simulink model "HANcoder_E407_TTA_Controller_v3_2"  (R2018b)
settings: Solver=FixedStepDiscrete  StartTime=0.0  StopTime=1  FixedStep=0.01  RelTol=1e-3
PreLoadFcn:
  | librarySetup
  | eval([bdroot,'_startup']) %Calling [modelName]_startup.m
undefined symbols (not defined in the file): A0, A1, A2, A3, A4, Backup_Board, basic_cycle_duration_bc0, basic_cycle_duration_bc1, comm_delay_estimation1, comm_delay_estimation2, COMM_Period, COMM_Phase1, COMM_Phase2, COMM_Phase_init1, COMM_Phase_init2, COMP_duration, CON2, CON4, Controller1_Board, Controller2_Board, Controller3_Board, D10, D12, D13, D8, D9, delta_a_set, delta_f_set, delta_max, delta_min, delta_precision, e_width, frequency_IRQ, HANtuneOverride, hardware_granularity, I_a, I_f, idle_time_init, Input_Gen_Board, LA_Clock_Gr, LA_COMM_dly, LA_COMM_Err, LA_E_Desync, LA_MEX_Flag, LA_Task_Act, m_v, Master_Role, matrix_cycle_duration, matrix_rows, max_desync, max_num_msgs_CAN1, max_num_msgs_CAN2, min_desync, OutControl1_ID, OutControl2_ID, OutEmulator_ID, R_al, R_ar, R_fl, R_fr ... (+80)
libraries: hdlsllib x434, HANcoder_STM32_Target x28, simulink x3, simulink_extras x1
(part 5 of 31)

== system HANcoder_E407_TTA_Controller_v3_2/HANcoder STM32 Target - E407-STM32 algorithm/TTA CAN System/CAN2 Recieve/RxID_CAN/SetValues_ID_CAN/CAN receive1 ==
  In1 : Inport
  Enabled Subsystem : Subsystem  TreatAsAtomicUnit=on
  S-Function : M-S-Function  FunctionName=sfcn_can_receive  Parameters=tsamp, canBus, outputNumber, dataType, byteOrder
  Out1 : Outport
  Out2 : Outport  Port=2
  Out3 : Outport  Port=3
  Out4 : Outport  Port=4
  Out5 : Outport  Port=5
  Out6 : Outport  Port=6
  Out7 : Outport  Port=7
  Out8 : Outport  Port=8
  Out9 : Outport  Port=9
  wires:
  S-Function/9 -> Enabled Subsystem/8(In8)
  S-Function/4 -> Enabled Subsystem/3(In3)
  S-Function/5 -> Enabled Subsystem/4(In4)
  S-Function/8 -> Enabled Subsystem/7(In7)
  S-Function/7 -> Enabled Subsystem/6(In6)
  S-Function/6 -> Enabled Subsystem/5(In5)
  Enabled Subsystem/8(Out8) -> Out9/1
  Enabled Subsystem/7(Out7) -> Out8/1
  Enabled Subsystem/6(Out6) -> Out7/1
  Enabled Subsystem/5(Out5) -> Out6/1
  Enabled Subsystem/4(Out4) -> Out5/1
  Enabled Subsystem/3(Out3) -> Out4/1
  Enabled Subsystem/2(Out2) -> Out3/1
  Enabled Subsystem/1(Out1) -> Out2/1
  S-Function/3 -> Enabled Subsystem/2(In2)
  S-Function/2 -> Enabled Subsystem/1(In1)
  S-Function/1 -> Out1/1, Enabled Subsystem/Enable
  In1/1 -> S-Function/1

== system HANcoder_E407_TTA_Controller_v3_2/HANcoder STM32 Target - E407-STM32 algorithm/TTA CAN System/CAN2 Recieve/RxID_CAN/Sync_ID_CAN/CAN receive1 ==
  In1 : Inport
  Enabled Subsystem : Subsystem  TreatAsAtomicUnit=on
  S-Function : M-S-Function  FunctionName=sfcn_can_receive  Parameters=tsamp, canBus, outputNumber, dataType, byteOrder
  Out1 : Outport
  Out2 : Outport  Port=2
  Out3 : Outport  Port=3
  Out4 : Outport  Port=4
  Out5 : Outport  Port=5
  Out6 : Outport  Port=6
  Out7 : Outport  Port=7
  Out8 : Outport  Port=8
  Out9 : Outport  Port=9
  wires:
  S-Function/9 -> Enabled Subsystem/8(In8)
  S-Function/4 -> Enabled Subsystem/3(In3)
  S-Function/5 -> Enabled Subsystem/4(In4)
  S-Function/8 -> Enabled Subsystem/7(In7)
  S-Function/7 -> Enabled Subsystem/6(In6)
  S-Function/6 -> Enabled Subsystem/5(In5)
  Enabled Subsystem/8(Out8) -> Out9/1
  Enabled Subsystem/7(Out7) -> Out8/1
  Enabled Subsystem/6(Out6) -> Out7/1
  Enabled Subsystem/5(Out5) -> Out6/1
  Enabled Subsystem/4(Out4) -> Out5/1
  Enabled Subsystem/3(Out3) -> Out4/1
  Enabled Subsystem/2(Out2) -> Out3/1
  Enabled Subsystem/1(Out1) -> Out2/1
  S-Function/3 -> Enabled Subsystem/2(In2)
  S-Function/2 -> Enabled Subsystem/1(In1)
  S-Function/1 -> Out1/1, Enabled Subsystem/Enable
  In1/1 -> S-Function/1

== system HANcoder_E407_TTA_Controller_v3_2/HANcoder STM32 Target - E407-STM32 algorithm/TTA CAN System/CAN2 Recieve/RxID_CAN/Vote1_ID_CAN/CAN receive1 ==
  In1 : Inport
  Enabled Subsystem : Subsystem  TreatAsAtomicUnit=on
  S-Function : M-S-Function  FunctionName=sfcn_can_receive  Parameters=tsamp, canBus, outputNumber, dataType, byteOrder
  Out1 : Outport
  Out2 : Outport  Port=2
  Out3 : Outport  Port=3
  Out4 : Outport  Port=4
  Out5 : Outport  Port=5
  Out6 : Outport  Port=6
  Out7 : Outport  Port=7
  Out8 : Outport  Port=8
  Out9 : Outport  Port=9
  wires:
  In1/1 -> S-Function/1
  S-Function/1 -> Enabled Subsystem/Enable, Out1/1
  S-Function/2 -> Enabled Subsystem/1(In1)
  S-Function/3 -> Enabled Subsystem/2(In2)
  Enabled Subsystem/1(Out1) -> Out2/1
  Enabled Subsystem/2(Out2) -> Out3/1
  Enabled Subsystem/3(Out3) -> Out4/1
  Enabled Subsystem/4(Out4) -> Out5/1
  Enabled Subsystem/5(Out5) -> Out6/1
  Enabled Subsystem/6(Out6) -> Out7/1
  Enabled Subsystem/7(Out7) -> Out8/1
  Enabled Subsystem/8(Out8) -> Out9/1
  S-Function/6 -> Enabled Subsystem/5(In5)
  S-Function/7 -> Enabled Subsystem/6(In6)
  S-Function/8 -> Enabled Subsystem/7(In7)
  S-Function/5 -> Enabled Subsystem/4(In4)
  S-Function/4 -> Enabled Subsystem/3(In3)
  S-Function/9 -> Enabled Subsystem/8(In8)

== system HANcoder_E407_TTA_Controller_v3_2/HANcoder STM32 Target - E407-STM32 algorithm/TTA CAN System/CAN2 Recieve/RxID_CAN/Vote2_ID_CAN/CAN receive1 ==
  In1 : Inport
  Enabled Subsystem : Subsystem  TreatAsAtomicUnit=on
  S-Function : M-S-Function  FunctionName=sfcn_can_receive  Parameters=tsamp, canBus, outputNumber, dataType, byteOrder
  Out1 : Outport
  Out2 : Outport  Port=2
  Out3 : Outport  Port=3
  Out4 : Outport  Port=4
  Out5 : Outport  Port=5
  Out6 : Outport  Port=6
  Out7 : Outport  Port=7
  Out8 : Outport  Port=8
  Out9 : Outport  Port=9
  wires:
  In1/1 -> S-Function/1
  S-Function/1 -> Enabled Subsystem/Enable, Out1/1
  S-Function/2 -> Enabled Subsystem/1(In1)
  S-Function/3 -> Enabled Subsystem/2(In2)
  Enabled Subsystem/1(Out1) -> Out2/1
  Enabled Subsystem/2(Out2) -> Out3/1
  Enabled Subsystem/3(Out3) -> Out4/1
  Enabled Subsystem/4(Out4) -> Out5/1
  Enabled Subsystem/5(Out5) -> Out6/1
  Enabled Subsystem/6(Out6) -> Out7/1
  Enabled Subsystem/7(Out7) -> Out8/1
  Enabled Subsystem/8(Out8) -> Out9/1
  S-Function/6 -> Enabled Subsystem/5(In5)
  S-Function/7 -> Enabled Subsystem/6(In6)
  S-Function/8 -> Enabled Subsystem/7(In7)
  S-Function/5 -> Enabled Subsystem/4(In4)
  S-Function/4 -> Enabled Subsystem/3(In3)
  S-Function/9 -> Enabled Subsystem/8(In8)

== system HANcoder_E407_TTA_Controller_v3_2/HANcoder STM32 Target - E407-STM32 algorithm/TTA CAN System/CAN2 Recieve/RxID_CAN/Vote3_ID_CAN/CAN receive1 ==
  In1 : Inport
  Enabled Subsystem : Subsystem  TreatAsAtomicUnit=on
  S-Function : M-S-Function  FunctionName=sfcn_can_receive  Parameters=tsamp, canBus, outputNumber, dataType, byteOrder
  Out1 : Outport
  Out2 : Outport  Port=2
  Out3 : Outport  Port=3
  Out4 : Outport  Port=4
  Out5 : Outport  Port=5
  Out6 : Outport  Port=6
  Out7 : Outport  Port=7
  Out8 : Outport  Port=8
  Out9 : Outport  Port=9
  wires:
  In1/1 -> S-Function/1
  S-Function/1 -> Enabled Subsystem/Enable, Out1/1
  S-Function/2 -> Enabled Subsystem/1(In1)
  S-Function/3 -> Enabled Subsystem/2(In2)
  Enabled Subsystem/1(Out1) -> Out2/1
  Enabled Subsystem/2(Out2) -> Out3/1
  Enabled Subsystem/3(Out3) -> Out4/1
  Enabled Subsystem/4(Out4) -> Out5/1
  Enabled Subsystem/5(Out5) -> Out6/1
  Enabled Subsystem/6(Out6) -> Out7/1
  Enabled Subsystem/7(Out7) -> Out8/1
  Enabled Subsystem/8(Out8) -> Out9/1
  S-Function/6 -> Enabled Subsystem/5(In5)
  S-Function/7 -> Enabled Subsystem/6(In6)
  S-Function/8 -> Enabled Subsystem/7(In7)
  S-Function/5 -> Enabled Subsystem/4(In4)
  S-Function/4 -> Enabled Subsystem/3(In3)
  S-Function/9 -> Enabled Subsystem/8(In8)

== system HANcoder_E407_TTA_Controller_v3_2/HANcoder STM32 Target - E407-STM32 algorithm/TTA CAN System/TTA System/Initialization/RoleID and Global Time init/Global Time Initialization Master ==
  note: Global Time Initialization
  Enable : EnablePort
  Board nr1 : Constant
  Cast : DataTypeConversion  OutDataTypeStr=uint16
  Cast1 : DataTypeConversion  OutDataTypeStr=uint8
  Data Store Write : DataStoreWrite  DataStoreName=Local_Ticks
  Data Store Write1 : DataStoreWrite  DataStoreName=basic_cycle_count
  Data Store Write3 : DataStoreWrite  DataStoreName=Master_ID
  Start : Constant  Value=0
  wires:
  Board nr1/1 -> Data Store Write3/1
  Start/1 -> Cast1/1, Cast/1
  Cast/1 -> Data Store Write/1
  Cast1/1 -> Data Store Write1/1

== system HANcoder_E407_TTA_Controller_v3_2/HANcoder STM32 Target - E407-STM32 algorithm/TTA CAN System/TTA System/Initialization/RoleID and Global Time init/Global Time Initialization Slave ==
  note: Sync has already been received, so we skip
      | the first comp tasks related to Update LT.
  note: Global Time Initialization
  note: Estimation of the Local Time when the message was sent
  Enable : EnablePort
  Bus Selector : BusSelector  OutputSignals=Buffer_1,Buffer_2,Buffer_3,Buffer_4,Buffer_5,Buffer_6,Buffer_7,Buffer_8
  Cast : DataTypeConversion  OutDataTypeStr=uint16
  Cast1 : DataTypeConversion  OutDataTypeStr=double
  Constant : Constant
  Constant1 : Constant  Value=COMM_Phase1
  Constant2 : Constant  Value=COMM_Phase2
  Constant3 : Constant  Value=TM_COMM_Sync
  Constant4 : Constant  Value=torque_precision
  Constant5 : Constant  Value=torque_precision
  Constant6 : Constant  Value=speed_precision
  Constant7 : Constant  Value=delta_precision
  Constant8 : Constant  Value=delta_precision
  Data Store Read : DataStoreRead  DataStoreName=New_Msg_Ready_CAN1
  Data Store Read1 : DataStoreRead  DataStoreName=Msg_Rx_CAN1
  Data Store Read2 : DataStoreRead  DataStoreName=Msg_Rx_CAN2
  Data Store Write : DataStoreWrite  DataStoreName=torque_fr_integral
  Data Store Write1 : DataStoreWrite  DataStoreName=Local_Ticks
  Data Store Write2 : DataStoreWrite  DataStoreName=basic_cycle_count
  Data Store Write3 : DataStoreWrite  DataStoreName=Master_ID
  Data Store Write4 : DataStoreWrite  Priority=10  DataStoreName=BC0_Sync_processed
  Data Store Write5 : DataStoreWrite  DataStoreName=torque_ar_integral
  Data Store Write6 : DataStoreWrite  DataStoreName=speed_integral
  Data Store Write7 : DataStoreWrite  DataStoreName=delta_f_est
  Data Store Write8 : DataStoreWrite  DataStoreName=delta_a_est
  Equal : RelationalOperator  Operator===  OutDataTypeStr=boolean  RndMeth=Simplest
  Multiply : Product
  Multiply1 : Product
  "SET1 " : Constant  Priority=9  OutDataTypeStr=boolean
  Sum : Sum  Inputs=+++
  Sum1 : Sum  Inputs=+++
  Switch : Switch  Criteria=u2 > Threshold
  Switch1 : Switch  Criteria=u2 > Threshold
  Terminator6 : Terminator
  Terminator7 : Terminator
  delay_estimation_1 : Constant  Value=comm_delay_estimation1
  delay_estimation_2 : Constant  Value=comm_delay_estimation2
  msg_decoding : Subsystem
  uint8_2float : Subsystem
  uint8_2float1 : Subsystem
  uint8_2float2 : Subsystem
  uint8_2float3 : Subsystem
  uint8_2float4 : Subsystem
  wires:
  Data Store Read/1 -> Equal/1
  Constant/1 -> Equal/2
  Bus Selector/5 -> uint8_2float3/2(value)  "<Buffer_5>"
  Bus Selector/8 -> Terminator7/1  "<Buffer_8>"
  Bus Selector/7 -> Terminator6/1  "<Buffer_7>"
  Bus Selector/6 -> uint8_2float4/2(value)  "<Buffer_6>"
  Switch/1 -> Bus Selector/1
  Bus Selector/1 -> msg_decoding/1(Msg_Temporal_Data)  "<Buffer_1>"
  Equal/1 -> Switch/2, [Rx_CAN1]
  Data Store Read1/1 -> Switch/1
  Data Store Read2/1 -> Switch/3
  "SET1 "/1 -> Data Store Write4/1
  Bus Selector/2 -> uint8_2float/2(value)  "<Buffer_2>"
  Bus Selector/3 -> uint8_2float1/2(value)  "<Buffer_3>"
  Bus Selector/4 -> uint8_2float2/2(value)  "<Buffer_4>"
  msg_decoding/1(basic_cycle) -> Data Store Write2/1  "Rx_init_bc"
  msg_decoding/3(board_id) -> Cast1/1  "Rx_init_id"
  Constant3/1 -> Sum/2, Sum1/2
  Constant2/1 -> Multiply1/1
  Constant1/1 -> Multiply/1
  delay_estimation_2/1 -> Sum1/3
  Sum/1 -> Switch1/1
  msg_decoding/2(msg_count) -> Multiply/2, Multiply1/2  "Rx_init_mc"
  Multiply/1 -> Sum/1
  Multiply1/1 -> Sum1/1
  Sum1/1 -> Switch1/3
  delay_estimation_1/1 -> Sum/3
  [Rx_CAN1] -> Switch1/2
  Switch1/1 -> Cast/1
  Cast/1 -> Data Store Write1/1  "Rx_init_LT"
  Cast1/1 -> Data Store Write3/1
  uint8_2float/1(decoded) -> Data Store Write/1
  Constant4/1 -> uint8_2float/1(precision)
  Constant5/1 -> uint8_2float1/1(precision)
  Constant6/1 -> uint8_2float2/1(precision)
  Constant7/1 -> uint8_2float3/1(precision)
  Constant8/1 -> uint8_2float4/1(precision)
  uint8_2float1/1(decoded) -> Data Store Write5/1
  uint8_2float2/1(decoded) -> Data Store Write6/1
  uint8_2float4/1(decoded) -> Data Store Write8/1
  uint8_2float3/1(decoded) -> Data Store Write7/1

== system HANcoder_E407_TTA_Controller_v3_2/HANcoder STM32 Target - E407-STM32 algorithm/TTA CAN System/TTA System/Matrix Cycle Manager/Backup Board Matrix Cycle/Backup board basic cycle 0 ==
  note: COMM - TW check
  note: COMP - TW check
  note: COMP - TW check
  note: COMP - TW check
  note: COMP - TW check
  note: Local Time still not updated
  note: Local Time still not updated
  note: Local Time still not updated
  note: Output Send_Message
      | Send: 1
      | Do not send: 0
  note: Output Receive_Message
      | Receive: 1
      | Do not receive: 0
  note: Output Receive_Message
      | Receive: 1
      | Do not receive: 0
  note: Output Send_Message
      | Send: 1
      | Do not send: 0
  Enable : EnablePort  PropagateVarSize=During execution
  AND{,1..2,15..19} (8 alike) : Logic  IconShape=distinctive  AllPortsSameDT=off  OutDataTypeStr=boolean
  COMM Task - Sync bc 0 : Subsystem
  COMP Task - Reset Board : Subsystem
  COMP Task - Reset Variables BC0 : Subsystem
  COMP Task - Sync bc0 check : Subsystem
  COMP Task - Update LT : Subsystem
  Constant : Constant  Value=TM_COMM_Sync
  Constant1 : Constant  Value=COMM_Period
  Constant{15..16,24,30} (4 alike) : Constant  Value=COMP_duration
  Constant17 : Constant  Value=TM_Update_LT
  Constant2 : Constant  Value=TM_Check_Sync
  Constant25 : Constant  Value=TM_Reset_Var
  Constant31 : Constant  Value=TM_Reset_Board
  Constant34 : Constant  Value=TM_Update_LT_2
  Data Store Memory11 : DataStoreMemory  DataStoreName=Msg_Rx  ReadBeforeWriteMsg=warning  WriteAfterWriteMsg=warning  WriteAfterReadMsg=warning  ShowAdditionalParam=off  OutDataTypeStr=Bus: msg_buffer_type
  Data Store Memory7 : DataStoreMemory  DataStoreName=Reset_Board  ReadBeforeWriteMsg=warning  WriteAfterWriteMsg=warning  WriteAfterReadMsg=warning  ShowAdditionalParam=off  OutDataTypeStr=boolean
  Data Store Memory8 : DataStoreMemory  DataStoreName=new_msg_Rx  ReadBeforeWriteMsg=warning  WriteAfterWriteMsg=warning  WriteAfterReadMsg=warning  ShowAdditionalParam=off
  Data Store Read11 : DataStoreRead  DataStoreName=BC0_Sync_processed
  Data Store Read6 : DataStoreRead  DataStoreName=BC0_Sync_processed
  Data Store Read7 : DataStoreRead  DataStoreName=BC0_Sync_processed
  Data Store Read8 : DataStoreRead  DataStoreName=Local_Ticks
  GreaterThan{,2,4,30,32} (5 alike) : RelationalOperator  OutDataTypeStr=boolean  RndMeth=Simplest
  GreaterThan{1,3,5,31,33} (5 alike) : RelationalOperator  Operator=<  OutDataTypeStr=boolean  RndMeth=Simplest
  NOT1 : Logic  Operator=NOT  IconShape=distinctive  AllPortsSameDT=off  OutDataTypeStr=boolean
  NOT2 : Logic  Operator=NOT  IconShape=distinctive  AllPortsSameDT=off  OutDataTypeStr=boolean
  NOT3 : Logic  Operator=NOT  IconShape=distinctive  AllPortsSameDT=off  OutDataTypeStr=boolean
  Sum{1..2,4,16..17} (5 alike) : Sum  Inputs=|++
  Send_Message_CAN1 : Outport  OutputWhenDisabled=reset  InitialOutput=0
  Send_Message_CAN2 : Outport  Port=2  OutputWhenDisabled=reset  InitialOutput=0
  Receive_Message_CAN1 : Outport  Port=3  OutputWhenDisabled=reset  InitialOutput=0
  Receive_Message_CAN2 : Outport  Port=4  OutputWhenDisabled=reset  InitialOutput=0
  wires:
  COMM Task - Sync bc 0/1(Send CAN1) -> [send_CAN1_Sync_bc0_TAG]
  COMM Task - Sync bc 0/2(Receive CAN1) -> [receive_CAN1_Sync_bc0_TAG]
  COMM Task - Sync bc 0/3(Send CAN2) -> [send_CAN2_Sync_bc0_TAG]
  COMM Task - Sync bc 0/4(Receive CAN2) -> [receive_CAN2_Sync_bc0_TAG]
  Constant1/1 -> Sum4/2
  Constant/1 -> COMP Task - Sync bc0 check/2(TM_COMM), COMM Task - Sync bc 0/1(Time Mark), Sum4/1, GreaterThan/2
  Sum4/1 -> GreaterThan1/2
  GreaterThan/1 -> AND/1
  GreaterThan1/1 -> AND/2
  AND/1 -> AND17/1
  GreaterThan3/1 -> AND1/2
  GreaterThan2/1 -> AND1/1
  Sum1/1 -> GreaterThan3/2
  Constant2/1 -> COMP Task - Sync bc0 check/1(Time_Mark), GreaterThan2/2, Sum1/1
  Constant15/1 -> Sum1/2
  Constant16/1 -> Sum2/2
  Constant17/1 -> COMP Task - Update LT/1(Time_Mark), Sum2/1, GreaterThan4/2
  Sum2/1 -> GreaterThan5/2
  GreaterThan4/1 -> AND2/1
  GreaterThan5/1 -> AND2/2
  GreaterThan31/1 -> AND15/2
  Sum16/1 -> GreaterThan31/2
  GreaterThan30/1 -> AND15/1
  Constant24/1 -> Sum16/2
  Constant25/1 -> COMP Task - Reset Variables BC0/1(Time_Mark), GreaterThan30/2, Sum16/1
  AND15/1 -> COMP Task - Reset Variables BC0/Enable
  Data Store Read8/1 -> GreaterThan32/1, GreaterThan33/1, GreaterThan31/1, GreaterThan30/1, GreaterThan4/1, GreaterThan5/1, GreaterThan2/1, GreaterThan3/1, GreaterThan/1, GreaterThan1/1
  AND16/1 -> COMP Task - Reset Board/Enable
  Constant31/1 -> COMP Task - Reset Board/1(Time_Mark), Sum17/1, GreaterThan32/2
  Constant30/1 -> Sum17/2
  GreaterThan32/1 -> AND16/1
  Sum17/1 -> GreaterThan33/2
  GreaterThan33/1 -> AND16/2
  Data Store Read11/1 -> NOT2/1
  NOT2/1 -> AND17/2
  AND17/1 -> COMM Task - Sync bc 0/Enable
  Data Store Read6/1 -> NOT1/1
  NOT1/1 -> AND18/2
  AND1/1 -> AND18/1
  AND18/1 -> COMP Task - Sync bc0 check/Enable
  Data Store Read7/1 -> NOT3/1
  NOT3/1 -> AND19/2
  AND2/1 -> AND19/1
  Constant34/1 -> COMP Task - Update LT/2(Time_Mark_2)
  AND19/1 -> COMP Task - Update LT/Enable
  [send_CAN1_Sync_bc0_TAG] -> Send_Message_CAN1/1
  [receive_CAN2_Sync_bc0_TAG] -> Receive_Message_CAN2/1
  [send_CAN2_Sync_bc0_TAG] -> Send_Message_CAN2/1
  [receive_CAN1_Sync_bc0_TAG] -> Receive_Message_CAN1/1

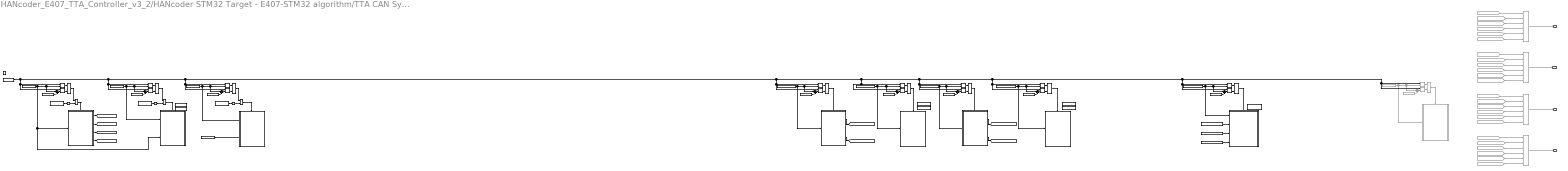
== system HANcoder_E407_TTA_Controller_v3_2/HANcoder STM32 Target - E407-STM32 algorithm/TTA CAN System/TTA System/Matrix Cycle Manager/Backup Board Matrix Cycle/Backup board basic cycle 1 ==
  note: Somehow get the values of the
      | third board for the comparisons
  note: Receive message condition
      | Sync Msg: Not Master and TM0
      | Vote Msg: Not # Node at TM#
  note: Send message condition
      | Sync Msg: Master and TM0
      | Vote Msg: Node# and TM#
  note: Output Send_Message
      | Send: 1
      | Do not send: 0
  note: Output Receive_Message
      | Receive: 1
      | Do not receive: 0
  note: Output Receive_Message
      | Receive: 1
      | Do not receive: 0
  note: Output Send_Message
      | Send: 1
      | Do not send: 0
  note: Send message condition
      | Sync Msg: Master and TM0
      | Vote Msg: Node# and TM#
  note: Receive message condition
      | Sync Msg: Not Master and TM0
      | Vote Msg: Not # Node at TM#
  note: COMM - TW check
  note: COMP - TW check
  note: COMM - TW check
  note: COMP - TW check
  note: Local Time still not updated
  note: COMP - TW check
  note: Local Time still not updated
  note: COMP - TW check
  note: COMM - TW check
  note: Local Time still not updated
  note: COMP - TW check
  note: COMP - TW check
  note: MEMBERSHIP FUNCTION
      |
      | Check which if there is a board faulty and which one
  Enable : EnablePort
  AND{,1..2,10..14,17..19} (11 alike) : Logic  IconShape=distinctive  AllPortsSameDT=off  OutDataTypeStr=boolean
  AND20 : Logic  Commented=on  IconShape=distinctive  AllPortsSameDT=off  OutDataTypeStr=boolean
  COMM Task - Output Control1 : Subsystem
  COMM Task - Output Control2 : Subsystem
  COMM Task - Sync bc 1 : Subsystem
  COMP Task - MF : Subsystem
  COMP Task - Reset Variables BC2 : Subsystem  Commented=on
  COMP Task - Rx_Output_Control1_Check : Subsystem
  COMP Task - Rx_Output_Control2_Check : Subsystem
  COMP Task - Sync bc1 check : Subsystem
  COMP Task - Update LT1 : Subsystem
  Constant : Constant  Value=TM_COMM_Sync
  Constant1 : Constant  Value=COMM_Period
  Constant10 : Constant  Value=COMM_Period
  Constant{2..3,11,13,22} (5 alike) : Constant  Value=COMP_duration
  Constant12 : Constant  Value=TM_Check_Output_Control2
  Constant14 : Constant  Value=TM_Memberschip_Function
  Constant15 : Constant  Commented=on  Value=COMP_duration
  Constant16 : Constant  Commented=on  Value=TM_Reset_Var_bc1
  Constant17 : Constant  Value=TM_Update_LT_2
  Constant23 : Constant  Value=TM_Check_Output_Control1
  Constant36 : Constant  Value=COMM_Period
  Constant37 : Constant  Value=TM_COMM_Output_Control2
  Constant38 : Constant  Value=TM_COMM_Output_Control1
  Constant39 : Constant  Value=TM_Memberschip_Function_2
  Constant4 : Constant  Value=TM_Update_LT
  Constant40 : Constant  Value=TM_Memberschip_Function_3
  Constant5 : Constant  Value=TM_Memberschip_Function_4
  Constant6 : Constant  Value=TM_Check_Sync
  Data Store Memory11 : DataStoreMemory  DataStoreName=Msg_Rx  ReadBeforeWriteMsg=warning  WriteAfterWriteMsg=warning  WriteAfterReadMsg=warning  ShowAdditionalParam=off  OutDataTypeStr=Bus: msg_buffer_type
  Data Store Memory19 : DataStoreMemory  DataStoreName=output_control1_rx  ReadBeforeWriteMsg=warning  WriteAfterWriteMsg=warning  WriteAfterReadMsg=warning  ShowAdditionalParam=off
  Data Store Memory47 : DataStoreMemory  DataStoreName=output_control1_msg  ReadBeforeWriteMsg=warning  WriteAfterWriteMsg=warning  WriteAfterReadMsg=warning  ShowAdditionalParam=off  OutDataTypeStr=Bus: msg_buffer_type
  Data Store Memory48 : DataStoreMemory  DataStoreName=output_control2_rx  ReadBeforeWriteMsg=warning  WriteAfterWriteMsg=warning  WriteAfterReadMsg=warning  ShowAdditionalParam=off
  Data Store Memory49 : DataStoreMemory  DataStoreName=output_control2_msg  ReadBeforeWriteMsg=warning  WriteAfterWriteMsg=warning  WriteAfterReadMsg=warning  ShowAdditionalParam=off  OutDataTypeStr=Bus: msg_buffer_type
  Data Store Memory50 : DataStoreMemory  DataStoreName=broken_board_ID  ReadBeforeWriteMsg=warning  WriteAfterWriteMsg=warning  WriteAfterReadMsg=warning  ShowAdditionalParam=off  OutDataTypeStr=uint8
  Data Store Memory8 : DataStoreMemory  DataStoreName=new_msg_Rx  ReadBeforeWriteMsg=warning  WriteAfterWriteMsg=warning  WriteAfterReadMsg=warning  ShowAdditionalParam=off
  Data Store Read1 : DataStoreRead  DataStoreName=Local_Ticks
  Data Store Read11 : DataStoreRead  DataStoreName=BC1_Sync_processed
  Data Store Read6 : DataStoreRead  DataStoreName=BC1_Sync_processed
  Data Store Read7 : DataStoreRead  DataStoreName=BC1_Sync_processed
  From160 : From  Commented=on  GotoTag=send_CAN1_Set_Values_bc1_TAG
  From161 : From  Commented=on  GotoTag=send_CAN1_Sensor_Values_bc1_TAG
  From162 : From  Commented=on  GotoTag=send_CAN1_Out_Control1_bc1_TAG
  From163 : From  Commented=on  GotoTag=send_CAN1_Out_Control2_bc1_TAG
  From164 : From  Commented=on  GotoTag=send_CAN1_Out_Emulator_bc1_TAG
  From165 : From  Commented=on  GotoTag=send_CAN2_Set_Values_bc1_TAG
  From166 : From  Commented=on  GotoTag=send_CAN2_Sensor_Values_bc1_TAG
  From167 : From  Commented=on  GotoTag=send_CAN2_Out_Control1_bc1_TAG
  From168 : From  Commented=on  GotoTag=send_CAN2_Out_Control2_bc1_TAG
  From169 : From  Commented=on  GotoTag=send_CAN2_Out_Emulator_bc1_TAG
  From17 : From  Commented=on  GotoTag=receive_CAN1_Sync_bc1_TAG
  From170 : From  Commented=on  GotoTag=receive_CAN1_Set_Values_bc1_TAG
  From171 : From  Commented=on  GotoTag=receive_CAN1_Sensor_Values_bc1_TAG
  From172 : From  Commented=on  GotoTag=receive_CAN1_Out_Control1_bc1_TAG
  From173 : From  Commented=on  GotoTag=receive_CAN1_Out_Control2_bc1_TAG
  From174 : From  Commented=on  GotoTag=receive_CAN1_Out_Emulator_bc1_TAG
  From175 : From  Commented=on  GotoTag=receive_CAN2_Set_Values_bc1_TAG
  From176 : From  Commented=on  GotoTag=receive_CAN2_Sensor_Values_bc1_TAG
  From177 : From  Commented=on  GotoTag=receive_CAN2_Out_Control1_bc1_TAG
  From178 : From  Commented=on  GotoTag=receive_CAN2_Out_Control2_bc1_TAG
  From179 : From  Commented=on  GotoTag=receive_CAN2_Out_Emulator_bc1_TAG
  From4 : From  Commented=on  GotoTag=send_CAN1_Sync_bc1_TAG
  From68 : From  Commented=on  GotoTag=receive_CAN2_Sync_bc1_TAG
  From82 : From  Commented=on  GotoTag=send_CAN2_Sync_bc1_TAG
  GreaterThan{,2,4,20,22,24,26,28} (8 alike) : RelationalOperator  OutDataTypeStr=boolean  RndMeth=Simplest
  GreaterThan{1,3,5,21,23,25,27,29} (8 alike) : RelationalOperator  Operator=<  OutDataTypeStr=boolean  RndMeth=Simplest
  GreaterThan34 : RelationalOperator  Commented=on  OutDataTypeStr=boolean  RndMeth=Simplest
  GreaterThan35 : RelationalOperator  Commented=on  Operator=<  OutDataTypeStr=boolean  RndMeth=Simplest
  NOT2 : Logic  Operator=NOT  IconShape=distinctive  AllPortsSameDT=off  OutDataTypeStr=boolean
  NOT4 : Logic  Operator=NOT  IconShape=distinctive  AllPortsSameDT=off  OutDataTypeStr=boolean
  NOT5 : Logic  Operator=NOT  IconShape=distinctive  AllPortsSameDT=off  OutDataTypeStr=boolean
  OR{1..4} (4 alike) : Logic  Commented=on  Operator=OR  Inputs=6  IconShape=distinctive  AllPortsSameDT=off  OutDataTypeStr=boolean
  Sum{1..2,4,11..15} (8 alike) : Sum  Inputs=|++
  Sum18 : Sum  Commented=on  Inputs=|++
  Send_Message_CAN1 : Outport  OutputWhenDisabled=reset  InitialOutput=0
  Send_Message_CAN2 : Outport  Port=2  OutputWhenDisabled=reset  InitialOutput=0
  Receive_Message_CAN1 : Outport  Port=3  OutputWhenDisabled=reset  InitialOutput=0
  Receive_Message_CAN2 : Outport  Port=4  OutputWhenDisabled=reset  InitialOutput=0
  wires:
  OR1/1 -> Send_Message_CAN1/1
  OR2/1 -> Receive_Message_CAN2/1
  OR4/1 -> Send_Message_CAN2/1
  OR3/1 -> Receive_Message_CAN1/1
  From4/1 -> OR1/1
  From160/1 -> OR1/2
  From161/1 -> OR1/3
  From162/1 -> OR1/4
  From163/1 -> OR1/5
  From164/1 -> OR1/6
  From82/1 -> OR4/1
  From165/1 -> OR4/2
  From166/1 -> OR4/3
  From167/1 -> OR4/4
  From168/1 -> OR4/5
  From169/1 -> OR4/6
  From17/1 -> OR3/1
  From170/1 -> OR3/2
  From171/1 -> OR3/3
  From172/1 -> OR3/4
  From174/1 -> OR3/6
  From173/1 -> OR3/5
  From68/1 -> OR2/1
  From175/1 -> OR2/2
  From177/1 -> OR2/4
  From176/1 -> OR2/3
  From178/1 -> OR2/5
  From179/1 -> OR2/6
  AND11/1 -> COMP Task - Rx_Output_Control1_Check/Enable
  AND12/1 -> COMM Task - Output Control2/Enable
  Constant1/1 -> Sum4/2
  COMM Task - Sync bc 1/1(Send CAN1) -> [send_CAN1_Sync_bc1_TAG]
  COMM Task - Sync bc 1/2(Receive CAN1) -> [receive_CAN1_Sync_bc1_TAG]
  COMM Task - Sync bc 1/4(Receive CAN2) -> [receive_CAN2_Sync_bc1_TAG]
  AND19/1 -> COMP Task - Update LT1/Enable
  Constant38/1 -> COMM Task - Output Control1/1(Time Mark), Sum12/1, GreaterThan24/2
  NOT2/1 -> AND18/2
  GreaterThan24/1 -> AND10/1
  GreaterThan22/1 -> AND12/1
  Sum14/1 -> GreaterThan27/2
  Data Store Read7/1 -> NOT5/1
  GreaterThan4/1 -> AND2/1
  AND18/1 -> COMP Task - Sync bc1 check/Enable
  AND1/1 -> AND18/1
  GreaterThan20/1 -> AND11/1
  Data Store Read11/1 -> NOT4/1
  AND13/1 -> COMP Task - Rx_Output_Control2_Check/Enable
  AND17/1 -> COMM Task - Sync bc 1/Enable
  GreaterThan25/1 -> AND10/2
  AND2/1 -> AND19/1
  Data Store Read6/1 -> NOT2/1
  NOT4/1 -> AND17/2
  GreaterThan23/1 -> AND12/2
  GreaterThan21/1 -> AND11/2
  GreaterThan1/1 -> AND/2
  GreaterThan/1 -> AND/1
  Constant37/1 -> Sum11/1, GreaterThan22/2, COMM Task - Output Control2/1(Time Mark)
  Constant12/1 -> COMP Task - Rx_Output_Control2_Check/1(Time_Mark), GreaterThan26/2, Sum14/1
  Constant/1 -> COMP Task - Sync bc1 check/2(TM_COMM), COMM Task - Sync bc 1/1(Time Mark), Sum4/1, GreaterThan/2
  GreaterThan26/1 -> AND13/1
  Constant11/1 -> Sum14/2
  Constant23/1 -> COMP Task - Rx_Output_Control1_Check/1(Time_Mark), GreaterThan20/2, Sum13/1
  Sum12/1 -> GreaterThan25/2
  Sum11/1 -> GreaterThan23/2
  Constant22/1 -> Sum13/2
  Constant10/1 -> Sum12/2
  AND/1 -> AND17/1
  Constant36/1 -> Sum11/2
  Constant3/1 -> Sum2/2
  AND10/1 -> COMM Task - Output Control1/Enable
  Constant4/1 -> COMP Task - Update LT1/1(Time_Mark), Sum2/1, GreaterThan4/2
  Sum4/1 -> GreaterThan1/2
  Sum13/1 -> GreaterThan21/2
  GreaterThan2/1 -> AND1/1
  GreaterThan3/1 -> AND1/2
  Constant2/1 -> Sum1/2
  Constant6/1 -> COMP Task - Sync bc1 check/1(Time_Mark), GreaterThan2/2, Sum1/1
  Sum1/1 -> GreaterThan3/2
  COMM Task - Sync bc 1/3(Send CAN2) -> [send_CAN2_Sync_bc1_TAG]
  GreaterThan27/1 -> AND13/2
  NOT5/1 -> AND19/2
  Sum2/1 -> GreaterThan5/2
  GreaterThan5/1 -> AND2/2
  COMM Task - Output Control1/1(Receive CAN1) -> [receive_CAN1_Out_Control1_bc1_TAG]
  COMM Task - Output Control1/2(Receive CAN2) -> [receive_CAN2_Out_Control1_bc1_TAG]
  COMM Task - Output Control2/1(Receive CAN1) -> [receive_CAN1_Out_Control2_bc1_TAG]
  COMM Task - Output Control2/2(Receive CAN2) -> [receive_CAN2_Out_Control2_bc1_TAG]
  GreaterThan35/1 -> AND20/2
  Constant16/1 -> COMP Task - Reset Variables BC2/1(Time_Mark), Sum18/1, GreaterThan34/2
  Constant15/1 -> Sum18/2
  Sum18/1 -> GreaterThan35/2
  GreaterThan34/1 -> AND20/1
  AND20/1 -> COMP Task - Reset Variables BC2/Enable
  Constant17/1 -> COMP Task - Update LT1/2(Time_Mark_2)
  Constant40/1 -> COMP Task - MF/3(Time_Mark_3)
  Constant14/1 -> COMP Task - MF/1(Time_Mark), Sum15/1, GreaterThan28/2
  Sum15/1 -> GreaterThan29/2
  GreaterThan29/1 -> AND14/2
  Data Store Read1/1 -> GreaterThan34/1, GreaterThan35/1, GreaterThan28/1, GreaterThan29/1, GreaterThan26/1, GreaterThan27/1, GreaterThan23/1, GreaterThan22/1, GreaterThan21/1, GreaterThan20/1, GreaterThan24/1, GreaterThan25/1, GreaterThan4/1, GreaterThan5/1, GreaterThan2/1, GreaterThan3/1, GreaterThan/1, GreaterThan1/1
  Constant13/1 -> Sum15/2
  AND14/1 -> COMP Task - MF/Enable
  GreaterThan28/1 -> AND14/1
  Constant39/1 -> COMP Task - MF/2(Time_Mark_2)
  Constant5/1 -> COMP Task - MF/4(Time_Mark_4)

== system HANcoder_E407_TTA_Controller_v3_2/HANcoder STM32 Target - E407-STM32 algorithm/TTA CAN System/TTA System/Matrix Cycle Manager/Backup Board Matrix Cycle/Matrix_Cycle_Observation_DEBUG ==
  Data Store Read : DataStoreRead  DataStoreName=Master_ID
  Data Store Read1 : DataStoreRead  DataStoreName=Role_ID
  Data Store Read10 : DataStoreRead  DataStoreName=BC1_Sync_processed
  Data Store Read11 : DataStoreRead  DataStoreName=Sync_bc0_missed_counter
  Data Store Read12 : DataStoreRead  DataStoreName=Sync_bc1_missed_counter
  Data Store Read13 : DataStoreRead  DataStoreName=Set_missed_counter
  Data Store Read14 : DataStoreRead  DataStoreName=Sensor_missed_counter
  Data Store Read15 : DataStoreRead  DataStoreName=Out1_missed_counter
  Data Store Read16 : DataStoreRead  DataStoreName=Out2_missed_counter
  Data Store Read2 : DataStoreRead  DataStoreName=BC0_Sync_processed
  Data Store Read3 : DataStoreRead  DataStoreName=Votes_count  DataStoreElements=Votes_count.First_Board#Votes_count.Second_Board#Votes_count.Third_Board
  Data Store Read4 : DataStoreRead  DataStoreName=Board1_error_counter
  Data Store Read5 : DataStoreRead  DataStoreName=Board2_error_counter
  Data Store Read6 : DataStoreRead  DataStoreName=Board3_error_counter
  Data Store Read7 : DataStoreRead  DataStoreName=BC0_Vote1_processed
  Data Store Read8 : DataStoreRead  DataStoreName=BC0_Vote2_processed
  Data Store Read9 : DataStoreRead  DataStoreName=BC0_Vote3_processed
  Terminator{,1..18} (19 alike) : Terminator
  wires:
  Data Store Read/1 -> Terminator1/1  "Master_ID_s"
  Data Store Read3/1 -> Terminator5/1  "votes_Board_1_DEBUG"
  Data Store Read3/2 -> Terminator6/1  "votes_Board_2_DEBUG"
  Data Store Read3/3 -> Terminator7/1  "votes_Board_3_DEBUG"
  Data Store Read4/1 -> Terminator8/1  "Board_1_error_counter_s"
  Data Store Read5/1 -> Terminator9/1  "Board_2_error_counter_s"
  Data Store Read6/1 -> Terminator10/1  "Board_3_error_counter_s"
  Data Store Read2/1 -> Terminator2/1  "BC0_sync_processed_s"
  Data Store Read7/1 -> Terminator3/1  "BC0_vote1_processed_s"
  Data Store Read8/1 -> Terminator4/1  "BC0_vote2_processed_s"
  Data Store Read9/1 -> Terminator11/1  "BC0_vote3_processed_s"
  Data Store Read10/1 -> Terminator12/1  "BC1_sync_processed_s"
  Data Store Read1/1 -> Terminator/1  "Role_ID_s"
  Data Store Read11/1 -> Terminator14/1  "sync_bc0_miss_counter_s"
  Data Store Read12/1 -> Terminator15/1  "sync_bc1_miss_counter_s"
  Data Store Read13/1 -> Terminator13/1  "set_miss_counter_s"
  Data Store Read14/1 -> Terminator17/1  "sensor_miss_counter_s"
  Data Store Read15/1 -> Terminator18/1  "out1_miss_counter_s"
  Data Store Read16/1 -> Terminator16/1  "out2_miss_counter_s"

== system HANcoder_E407_TTA_Controller_v3_2/HANcoder STM32 Target - E407-STM32 algorithm/TTA CAN System/TTA System/Matrix Cycle Manager/Backup Board Matrix Cycle/msg_count_DEBUG observer ==
  Data Store Read24 : DataStoreRead  DataStoreName=msg_count_DEBUG
  Terminator : Terminator
  wires:
  Data Store Read24/1 -> Terminator/1  "msg_count_DEBUG_s"

== system HANcoder_E407_TTA_Controller_v3_2/HANcoder STM32 Target - E407-STM32 algorithm/TTA CAN System/TTA System/Matrix Cycle Manager/Controller Matrix Cycle/Matrix_Cycle_Observation_DEBUG ==
  Data Store Read : DataStoreRead  DataStoreName=Master_ID
  Data Store Read1 : DataStoreRead  DataStoreName=Role_ID
  Data Store Read10 : DataStoreRead  DataStoreName=BC1_Sync_processed
  Data Store Read11 : DataStoreRead  DataStoreName=Sync_bc0_missed_counter
  Data Store Read12 : DataStoreRead  DataStoreName=Sync_bc1_missed_counter
  Data Store Read13 : DataStoreRead  DataStoreName=Set_missed_counter
  Data Store Read14 : DataStoreRead  DataStoreName=Sensor_missed_counter
  Data Store Read15 : DataStoreRead  DataStoreName=Out1_missed_counter
  Data Store Read16 : DataStoreRead  DataStoreName=Out2_missed_counter
  Data Store Read2 : DataStoreRead  DataStoreName=BC0_Sync_processed
  Data Store Read3 : DataStoreRead  DataStoreName=Votes_count  DataStoreElements=Votes_count.First_Board#Votes_count.Second_Board#Votes_count.Third_Board
  Data Store Read4 : DataStoreRead  DataStoreName=Board1_error_counter
  Data Store Read5 : DataStoreRead  DataStoreName=Board2_error_counter
  Data Store Read6 : DataStoreRead  DataStoreName=Board3_error_counter
  Data Store Read7 : DataStoreRead  DataStoreName=BC0_Vote1_processed
  Data Store Read8 : DataStoreRead  DataStoreName=BC0_Vote2_processed
  Data Store Read9 : DataStoreRead  DataStoreName=BC0_Vote3_processed
  Terminator{,1..18} (19 alike) : Terminator
  wires:
  Data Store Read/1 -> Terminator1/1  "Master_ID_s"
  Data Store Read3/1 -> Terminator5/1  "votes_Board_1_DEBUG"
  Data Store Read3/2 -> Terminator6/1  "votes_Board_2_DEBUG"
  Data Store Read3/3 -> Terminator7/1  "votes_Board_3_DEBUG"
  Data Store Read4/1 -> Terminator8/1  "Board_1_error_counter_s"
  Data Store Read5/1 -> Terminator9/1  "Board_2_error_counter_s"
  Data Store Read6/1 -> Terminator10/1  "Board_3_error_counter_s"
  Data Store Read2/1 -> Terminator2/1  "BC0_sync_processed_s"
  Data Store Read7/1 -> Terminator3/1  "BC0_vote1_processed_s"
  Data Store Read8/1 -> Terminator4/1  "BC0_vote2_processed_s"
  Data Store Read9/1 -> Terminator11/1  "BC0_vote3_processed_s"
  Data Store Read10/1 -> Terminator12/1  "BC1_sync_processed_s"
  Data Store Read1/1 -> Terminator/1  "Role_ID_s"
  Data Store Read11/1 -> Terminator14/1  "sync_bc0_miss_counter_s"
  Data Store Read12/1 -> Terminator15/1  "sync_bc1_miss_counter_s"
  Data Store Read13/1 -> Terminator13/1  "set_miss_counter_s"
  Data Store Read14/1 -> Terminator17/1  "sensor_miss_counter_s"
  Data Store Read15/1 -> Terminator18/1  "out1_miss_counter_s"
  Data Store Read16/1 -> Terminator16/1  "out2_miss_counter_s"

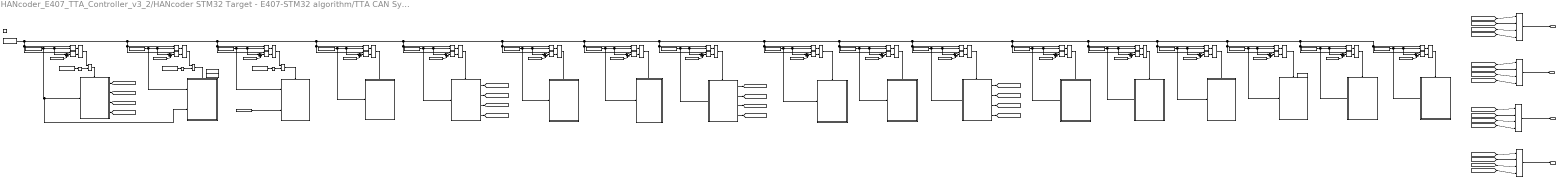
== system HANcoder_E407_TTA_Controller_v3_2/HANcoder STM32 Target - E407-STM32 algorithm/TTA CAN System/TTA System/Matrix Cycle Manager/Controller Matrix Cycle/controller basic cycle 0 ==
  note: Output Send_Message
      | Send: 1
      | Do not send: 0
  note: Send message condition
      | Sync Msg: Master and TM0
      | Vote Msg: Node# and TM#
  note: Receive message condition
      | Sync Msg: Not Master and TM0
      | Vote Msg: Not # Node at TM#
  note: Receive message condition
      | Sync Msg: Not Master and TM0
      | Vote Msg: Not # Node at TM#
  note: Output Receive_Message
      | Receive: 1
      | Do not receive: 0
  note: Output Send_Message
      | Send: 1
      | Do not send: 0
  note: Output Receive_Message
      | Receive: 1
      | Do not receive: 0
  note: Send message condition
      | Sync Msg: Master and TM0
      | Vote Msg: Node# and TM#
  note: COMM - TW check
  note: COMP - TW check
  note: COMP - TW check
  note: COMP - TW check
  note: COMM - TW check
  note: COMP - TW check
  note: COMP - TW check
  note: COMM - TW check
  note: COMP - TW check
  note: COMP - TW check
  note: COMM - TW check
  note: COMP - TW check
  note: COMP - TW check
  note: COMP - TW check
  note: COMP - TW check
  note: COMP - TW check
  note: COMP - TW check
  note: Local Time still not updated
  note: Local Time still not updated
  note: Local Time still not updated
  Enable : EnablePort  PropagateVarSize=During execution
  AND{,1..19} (20 alike) : Logic  IconShape=distinctive  AllPortsSameDT=off  OutDataTypeStr=boolean
  COMM Task - Sync bc 0 : Subsystem
  COMM Task - Vote1 : Subsystem
  COMM Task - Vote2 : Subsystem
  COMM Task - Vote3 : Subsystem
  COMP Task - Check Timeouts : Subsystem
  COMP Task - New Master : Subsystem
  COMP Task - Reset Board : Subsystem
  COMP Task - Reset Variables BC0 : Subsystem
  COMP Task - Sync bc0 check : Subsystem
  COMP Task - Update LT : Subsystem
  COMP Task - Vote Decision : Subsystem
  COMP Task - Vote1 Count : Subsystem
  COMP Task - Vote1 check : Subsystem
  COMP Task - Vote2 Count : Subsystem
  COMP Task - Vote2 check : Subsystem
  COMP Task - Vote3 Count : Subsystem
  COMP Task - Vote3 check : Subsystem
  Constant : Constant  Value=TM_COMM_Sync
  Constant{1,4,10,29} (4 alike) : Constant  Value=COMM_Period
  Constant{5,7,11,13,15..16,18,20,22,24,26,30,32} (13 alike) : Constant  Value=COMP_duration
  Constant12 : Constant  Value=TM_Check_TOuts
  Constant14 : Constant  Value=TM_New_Master
  Constant17 : Constant  Value=TM_Update_LT
  Constant19 : Constant  Value=TM_Vote_Dec
  Constant2 : Constant  Value=TM_Check_Sync
  Constant21 : Constant  Value=TM_Count_Vote1
  Constant23 : Constant  Value=TM_Check_Vote3
  Constant25 : Constant  Value=TM_Reset_Var
  Constant27 : Constant  Value=TM_Count_Vote2
  Constant28 : Constant  Value=TM_COMM_Vote2
  Constant3 : Constant  Value=TM_COMM_Vote1
  Constant31 : Constant  Value=TM_Reset_Board
  Constant33 : Constant  Value=TM_Check_Vote2
  Constant34 : Constant  Value=TM_Update_LT_2
  Constant6 : Constant  Value=TM_Check_Vote1
  Constant8 : Constant  Value=TM_Count_Vote3
  Constant9 : Constant  Value=TM_COMM_Vote3
  Data Store Memory11 : DataStoreMemory  DataStoreName=Msg_Rx  ReadBeforeWriteMsg=warning  WriteAfterWriteMsg=warning  WriteAfterReadMsg=warning  ShowAdditionalParam=off  OutDataTypeStr=Bus: msg_buffer_type
  Data Store Memory7 : DataStoreMemory  DataStoreName=Reset_Board  ReadBeforeWriteMsg=warning  WriteAfterWriteMsg=warning  WriteAfterReadMsg=warning  ShowAdditionalParam=off  OutDataTypeStr=boolean
  Data Store Memory8 : DataStoreMemory  DataStoreName=new_msg_Rx  ReadBeforeWriteMsg=warning  WriteAfterWriteMsg=warning  WriteAfterReadMsg=warning  ShowAdditionalParam=off
  Data Store Read11 : DataStoreRead  DataStoreName=BC0_Sync_processed
  Data Store Read6 : DataStoreRead  DataStoreName=BC0_Sync_processed
  Data Store Read7 : DataStoreRead  DataStoreName=BC0_Sync_processed
  Data Store Read8 : DataStoreRead  DataStoreName=Local_Ticks
  GreaterThan{,2,4,6,8,10,12,14,16,18,20,22,24,26,28,30,32} (17 alike) : RelationalOperator  OutDataTypeStr=boolean  RndMeth=Simplest
  GreaterThan{1,3,5,7,9,11,13,15,17,19,21,23,25,27,29,31,33} (17 alike) : RelationalOperator  Operator=<  OutDataTypeStr=boolean  RndMeth=Simplest
  NOT1 : Logic  Operator=NOT  IconShape=distinctive  AllPortsSameDT=off  OutDataTypeStr=boolean
  NOT2 : Logic  Operator=NOT  IconShape=distinctive  AllPortsSameDT=off  OutDataTypeStr=boolean
  NOT3 : Logic  Operator=NOT  IconShape=distinctive  AllPortsSameDT=off  OutDataTypeStr=boolean
  OR{1..4} (4 alike) : Logic  Operator=OR  Inputs=4  IconShape=distinctive  AllPortsSameDT=off  OutDataTypeStr=boolean
  Sum{1..17} (17 alike) : Sum  Inputs=|++
  Send_Message_CAN1 : Outport  OutputWhenDisabled=reset  InitialOutput=0
  Send_Message_CAN2 : Outport  Port=2  OutputWhenDisabled=reset  InitialOutput=0
  Receive_Message_CAN1 : Outport  Port=3  OutputWhenDisabled=reset  InitialOutput=0
  Receive_Message_CAN2 : Outport  Port=4  OutputWhenDisabled=reset  InitialOutput=0
  wires:
  OR1/1 -> Send_Message_CAN1/1
  [receive_CAN2_Sync_bc0_TAG] -> OR3/1
  [receive_CAN2_Vote3_bc0_TAG] -> OR3/4
  [receive_CAN2_Vote1_bc0_TAG] -> OR3/2
  [receive_CAN2_Vote2_bc0_TAG] -> OR3/3
  OR3/1 -> Receive_Message_CAN2/1
  [receive_CAN1_Sync_bc0_TAG] -> OR2/1
  [receive_CAN1_Vote1_bc0_TAG] -> OR2/2
  [receive_CAN1_Vote2_bc0_TAG] -> OR2/3
  [receive_CAN1_Vote3_bc0_TAG] -> OR2/4
  OR2/1 -> Receive_Message_CAN1/1
  [send_CAN2_Sync_bc0_TAG] -> OR4/1
  [send_CAN2_Vote1_bc0_TAG] -> OR4/2
  [send_CAN2_Vote2_bc0_TAG] -> OR4/3
  [send_CAN2_Vote3_bc0_TAG] -> OR4/4
  [send_CAN1_Sync_bc0_TAG] -> OR1/1
  [send_CAN1_Vote1_bc0_TAG] -> OR1/2
  [send_CAN1_Vote2_bc0_TAG] -> OR1/3
  [send_CAN1_Vote3_bc0_TAG] -> OR1/4
  OR4/1 -> Send_Message_CAN2/1
  COMM Task - Sync bc 0/1(Send CAN1) -> [send_CAN1_Sync_bc0_TAG]
  COMM Task - Sync bc 0/2(Receive CAN1) -> [receive_CAN1_Sync_bc0_TAG]
  COMM Task - Sync bc 0/3(Send CAN2) -> [send_CAN2_Sync_bc0_TAG]
  COMM Task - Sync bc 0/4(Receive CAN2) -> [receive_CAN2_Sync_bc0_TAG]
  Constant1/1 -> Sum4/2
  Constant/1 -> COMP Task - Sync bc0 check/2(TM_COMM), COMM Task - Sync bc 0/1(Time Mark), Sum4/1, GreaterThan/2
  Sum4/1 -> GreaterThan1/2
  GreaterThan/1 -> AND/1
  GreaterThan1/1 -> AND/2
  AND/1 -> AND17/1
  GreaterThan3/1 -> AND1/2
  GreaterThan2/1 -> AND1/1
  Sum1/1 -> GreaterThan3/2
  Constant2/1 -> COMP Task - Sync bc0 check/1(Time_Mark), GreaterThan2/2, Sum1/1
  Constant15/1 -> Sum1/2
  Constant16/1 -> Sum2/2
  Constant17/1 -> COMP Task - Update LT/1(Time_Mark), Sum2/1, GreaterThan4/2
  Sum2/1 -> GreaterThan5/2
  GreaterThan4/1 -> AND2/1
  GreaterThan5/1 -> AND2/2
  AND3/1 -> COMP Task - Vote Decision/Enable
  GreaterThan7/1 -> AND3/2
  GreaterThan6/1 -> AND3/1
  Sum3/1 -> GreaterThan7/2
  Constant19/1 -> COMP Task - Vote Decision/1(Time Mark), GreaterThan6/2, Sum3/1
  Constant18/1 -> Sum3/2
  COMM Task - Vote1/1(Send CAN1) -> [send_CAN1_Vote1_bc0_TAG]
  COMM Task - Vote1/2(Receive CAN1) -> [receive_CAN1_Vote1_bc0_TAG]
  COMM Task - Vote1/3(Send CAN2) -> [send_CAN2_Vote1_bc0_TAG]
  COMM Task - Vote1/4(Receive CAN2) -> [receive_CAN2_Vote1_bc0_TAG]
  GreaterThan9/1 -> AND4/2
  GreaterThan8/1 -> AND4/1
  Sum5/1 -> GreaterThan9/2
  Constant4/1 -> Sum5/2
  AND4/1 -> COMM Task - Vote1/Enable
  Constant3/1 -> COMM Task - Vote1/1(Time Mark), Sum5/1, GreaterThan8/2
  GreaterThan11/1 -> AND5/2
  Sum6/1 -> GreaterThan11/2
  GreaterThan10/1 -> AND5/1
  Constant5/1 -> Sum6/2
  Constant6/1 -> COMP Task - Vote1 check/1(Time_Mark), GreaterThan10/2, Sum6/1
  AND5/1 -> COMP Task - Vote1 check/Enable
  AND6/1 -> COMP Task - Vote1 Count/Enable
  Constant21/1 -> COMP Task - Vote1 Count/1(Time Mark), Sum7/1, GreaterThan12/2
  Constant20/1 -> Sum7/2
  GreaterThan12/1 -> AND6/1
  Sum7/1 -> GreaterThan13/2
  GreaterThan13/1 -> AND6/2
  GreaterThan17/1 -> AND9/2
  Sum10/1 -> GreaterThan17/2
  GreaterThan16/1 -> AND9/1
  Constant26/1 -> Sum10/2
  Constant27/1 -> COMP Task - Vote2 Count/1(Time Mark), GreaterThan16/2, Sum10/1
  AND9/1 -> COMP Task - Vote2 Count/Enable
  Constant33/1 -> COMP Task - Vote2 check/1(Time_Mark), Sum9/1, GreaterThan14/2
  Constant32/1 -> Sum9/2
  GreaterThan14/1 -> AND8/1
  Sum9/1 -> GreaterThan15/2
  GreaterThan15/1 -> AND8/2
  Constant28/1 -> COMM Task - Vote2/1(Time Mark), GreaterThan18/2, Sum8/1
  AND7/1 -> COMM Task - Vote2/Enable
  Constant29/1 -> Sum8/2
  Sum8/1 -> GreaterThan19/2
  GreaterThan18/1 -> AND7/1
  GreaterThan19/1 -> AND7/2
  COMM Task - Vote2/1(Send CAN1) -> [send_CAN1_Vote2_bc0_TAG]
  COMM Task - Vote2/2(Receive CAN1) -> [receive_CAN1_Vote2_bc0_TAG]
  COMM Task - Vote2/3(Send CAN2) -> [send_CAN2_Vote2_bc0_TAG]
  AND8/1 -> COMP Task - Vote2 check/Enable
  GreaterThan25/1 -> AND10/2
  GreaterThan24/1 -> AND10/1
  Sum12/1 -> GreaterThan25/2
  Constant10/1 -> Sum12/2
  Constant9/1 -> COMM Task - Vote3/1(Time Mark), Sum12/1, GreaterThan24/2
  GreaterThan21/1 -> AND11/2
  Sum13/1 -> GreaterThan21/2
  GreaterThan20/1 -> AND11/1
  Constant22/1 -> Sum13/2
  Constant23/1 -> COMP Task - Vote3 check/1(Time_Mark), GreaterThan20/2, Sum13/1
  AND12/1 -> COMP Task - Vote3 Count/Enable
  Constant8/1 -> COMP Task - Vote3 Count/1(Time Mark), Sum11/1, GreaterThan22/2
  Constant7/1 -> Sum11/2
  GreaterThan22/1 -> AND12/1
  Sum11/1 -> GreaterThan23/2
  GreaterThan23/1 -> AND12/2
  COMM Task - Vote3/1(Send CAN1) -> [send_CAN1_Vote3_bc0_TAG]
  COMM Task - Vote3/2(Receive CAN1) -> [receive_CAN1_Vote3_bc0_TAG]
  COMM Task - Vote3/3(Send CAN2) -> [send_CAN2_Vote3_bc0_TAG]
  COMM Task - Vote3/4(Receive CAN2) -> [receive_CAN2_Vote3_bc0_TAG]
  AND10/1 -> COMM Task - Vote3/Enable
  AND11/1 -> COMP Task - Vote3 check/Enable
  GreaterThan27/1 -> AND13/2
  Sum14/1 -> GreaterThan27/2
  GreaterThan26/1 -> AND13/1
  Constant11/1 -> Sum14/2
  Constant12/1 -> COMP Task - Check Timeouts/1(Time_Mark), GreaterThan26/2, Sum14/1
  AND13/1 -> COMP Task - Check Timeouts/Enable
  AND14/1 -> COMP Task - New Master/Enable
  Constant14/1 -> COMP Task - New Master/1(Time_Mark), Sum15/1, GreaterThan28/2
  Constant13/1 -> Sum15/2
  GreaterThan28/1 -> AND14/1
  Sum15/1 -> GreaterThan29/2
  GreaterThan29/1 -> AND14/2
  GreaterThan31/1 -> AND15/2
  Sum16/1 -> GreaterThan31/2
  GreaterThan30/1 -> AND15/1
  Constant24/1 -> Sum16/2
  Constant25/1 -> COMP Task - Reset Variables BC0/1(Time_Mark), GreaterThan30/2, Sum16/1
  AND15/1 -> COMP Task - Reset Variables BC0/Enable
  Data Store Read8/1 -> GreaterThan21/1, GreaterThan20/1, GreaterThan22/1, GreaterThan23/1, GreaterThan32/1, GreaterThan33/1, GreaterThan31/1, GreaterThan30/1, GreaterThan28/1, GreaterThan29/1, GreaterThan27/1, GreaterThan26/1, GreaterThan25/1, GreaterThan24/1, GreaterThan17/1, GreaterThan16/1, GreaterThan14/1, GreaterThan15/1, GreaterThan18/1, GreaterThan19/1, GreaterThan12/1, GreaterThan13/1, GreaterThan11/1, GreaterThan10/1, GreaterThan9/1, GreaterThan8/1, GreaterThan6/1, GreaterThan7/1, GreaterThan4/1, GreaterThan5/1, GreaterThan2/1, GreaterThan3/1, GreaterThan/1, GreaterThan1/1
  AND16/1 -> COMP Task - Reset Board/Enable
  Constant31/1 -> COMP Task - Reset Board/1(Time_Mark), Sum17/1, GreaterThan32/2
  Constant30/1 -> Sum17/2
  GreaterThan32/1 -> AND16/1
  Sum17/1 -> GreaterThan33/2
  GreaterThan33/1 -> AND16/2
  Data Store Read11/1 -> NOT2/1
  NOT2/1 -> AND17/2
  AND17/1 -> COMM Task - Sync bc 0/Enable
  Data Store Read6/1 -> NOT1/1
  NOT1/1 -> AND18/2
  AND1/1 -> AND18/1
  AND18/1 -> COMP Task - Sync bc0 check/Enable
  Data Store Read7/1 -> NOT3/1
  NOT3/1 -> AND19/2
  AND2/1 -> AND19/1
  AND19/1 -> COMP Task - Update LT/Enable
  COMM Task - Vote2/4(Receive CAN2) -> [receive_CAN2_Vote2_bc0_TAG]
  Constant34/1 -> COMP Task - Update LT/2(Time_Mark_2)
